simulink model "stabilitySimulation"  (R2017a)
settings: Solver=VariableStepAuto  StartTime=0.0  StopTime=100  RelTol=1e-3
undefined symbols (not defined in the file): b, k0, k1, M
libraries: simulink x4
settings Model: Creator=HP  LastModifiedBy=HP

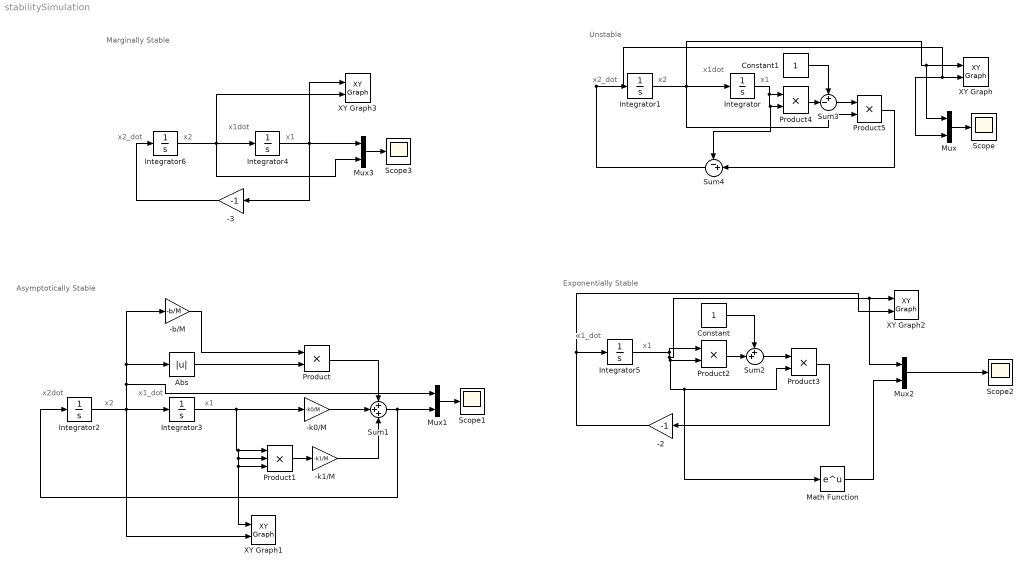
== system stabilitySimulation ==
  note: Exponentially Stable
  note: Asymptotically Stable
  note: Unstable
  note: x1dot
  note: x2_dot
  note: x2
  note: x1_dot
  note: x1
  note: x2dot
  note: x1
  note: x2
  note: x1_dot
  note: x1
  note: Marginally Stable
  note: x1dot
  note: x2_dot
  note: x1
  note: x2
  -2 : Gain  Gain=-1
  -3 : Gain  Gain=-1
  -b/M : Gain  Gain=-b/M
  -k0/M : Gain  Gain=-k0/M
  -k1/M : Gain  Gain=-k1/M
  Abs : Abs
  Constant : Constant
  Constant1 : Constant
  Integrator{,1..6} (7 alike) : Integrator  InitialCondition=1
  Math Function : Math  SaturateOnIntegerOverflow=on
  Mux{,1..3} (4 alike) : Mux  Inputs=2
  Product{,2..5} (5 alike) : Product
  Product1 : Product  Inputs=3
  Scope{,1..3} (4 alike) : Scope
  Sum1 : Sum  Inputs=+++
  Sum2 : Sum  Inputs=++|
  Sum3 : Sum  Inputs=+-|
  Sum4 : Sum  Inputs=-+|
  XY Graph{,1..3} (4 alike) : simulink/Sinks/XY Graph  xmin=-2.5  xmax=2.5  ymin=-2.5  ymax=2.5  st=-1
  wires:
  Integrator1/1 -> Product5/2, Mux/1, XY Graph/1, Integrator/1
  Abs/1 -> Product/2
  -b/M/1 -> Product/1
  Integrator3/1 -> XY Graph1/1, Product1/3, Product1/2, Product1/1, -k0/M/1
  Product1/1 -> -k1/M/1
  Product/1 -> Sum1/1
  -k0/M/1 -> Sum1/2
  -k1/M/1 -> Sum1/3
  Mux/1 -> Scope/1
  Mux1/1 -> Scope1/1
  Sum1/1 -> Mux1/2, Integrator2/1
  Integrator2/1 -> XY Graph1/2, Mux1/1, -b/M/1, Abs/1, Integrator3/1
  Mux2/1 -> Scope2/1
  Integrator5/1 -> Product2/1, Mux2/1, XY Graph2/1, Math Function/1, Product3/2, Product2/2
  Product2/1 -> Sum2/2
  Constant/1 -> Sum2/1
  Sum2/1 -> Product3/1
  Product3/1 -> -2/1
  -2/1 -> XY Graph2/2, Integrator5/1
  Math Function/1 -> Mux2/2
  -3/1 -> Integrator6/1
  Mux3/1 -> Scope3/1
  Integrator6/1 -> Integrator4/1, Mux3/2, XY Graph3/2
  Integrator4/1 -> -3/1, Mux3/1, XY Graph3/1
  Integrator/1 -> Sum4/1, Product4/2, Product4/1
  Product4/1 -> Sum3/2
  Constant1/1 -> Sum3/1
  Sum3/1 -> Product5/1
  Product5/1 -> Sum4/2
  Sum4/1 -> XY Graph/2, Mux/2, Integrator1/1
